simulink model "gold_mine"  (R2024b)
settings: Solver=VariableStepAuto  StartTime=0.0  StopTime=1  RelTol=1e-3
values from neighbouring files (symbols this model uses):
  Capital_expenditure = plan_4mt(:, 14)    [DCF_Model_for_Mining_Inv.m]
  discount_rate = 0.10    (= 0.1)    [DCF_Model_for_Mining_Inv.m]
  Gold_price = gold_price_matrix    [DCF_Model_for_Mining_Inv.m]
  inflation = 0.02    [DCF_Model_for_Mining_Inv.m]
  Mill1 = plan_4mt(:, 3)    [DCF_Model_for_Mining_Inv.m]
  Mill_Au_GRADE = plan_4mt(:, 4)    [DCF_Model_for_Mining_Inv.m]
  mining_cost_initial = 3.10    (= 3.1)    [DCF_Model_for_Mining_Inv.m]
  Period = plan_4mt(:, 1)    [DCF_Model_for_Mining_Inv.m]
  Recovery_rate = plan_4mt(:, 8)    [DCF_Model_for_Mining_Inv.m]
  Tax_and_royalty = plan_4mt(:, 17)    [DCF_Model_for_Mining_Inv.m]
  Tonnes = plan_4mt(:, 2)    [DCF_Model_for_Mining_Inv.m]
  Unit_processing_cost = plan_4mt(:, 10)    [DCF_Model_for_Mining_Inv.m]
undefined symbols (not defined in the file or in its folder): Stockpile_in, Stockpile_out, Waste
settings Model: Creator=eerolindholm  LastModifiedBy=eerolindholm

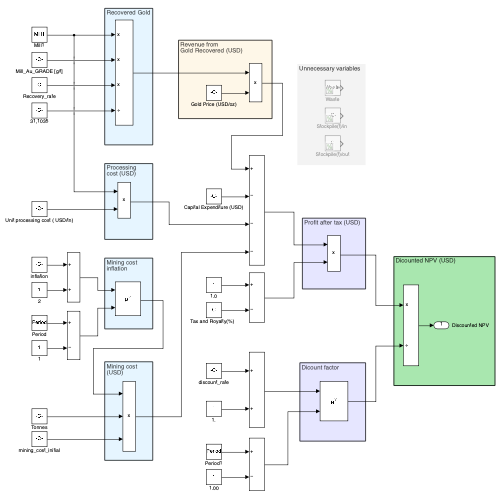
[thumbnail: Simulink's stored preview of the top-level diagram]
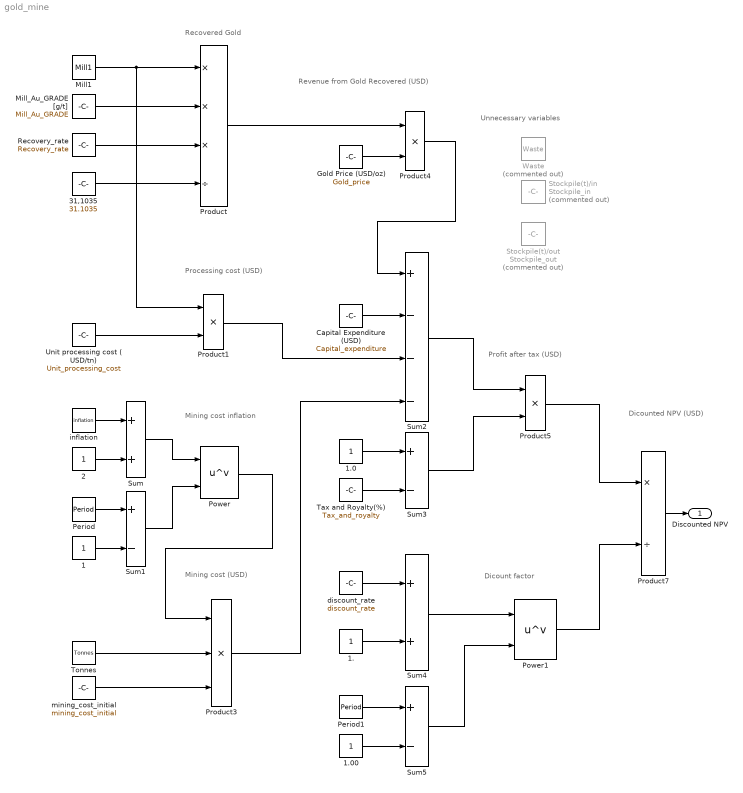
== system gold_mine ==
  note: Unnecessary variables
  note: Dicounted NPV (USD)
  note: Dicount factor
  note: Profit after tax (USD)
  note: Revenue from
      | Gold Recovered (USD)
  note: Mining cost
      | inflation
  note: Recovered Gold
  note: Processing
      | cost (USD)
  note: Mining cost
      | (USD)
  1 : Constant
  1. : Constant
  1.0 : Constant
  1.00 : Constant
  2 : Constant
  31,1035 : Constant  Value=31.1035
  Capital Expenditure (USD) : Constant  Value=Capital_expenditure
  Gold Price (USD/oz) : Constant  Value=Gold_price
  Mill1 : Constant  Value=Mill1
  Mill_Au_GRADE [g/t] : Constant  Value=Mill_Au_GRADE
  Period : Constant  Value=Period
  Period1 : Constant  Value=Period
  Power : Math  Operator=pow
  Power1 : Math  Operator=pow
  Product : Product  Inputs=***/
  Product1 : Product  Inputs=**
  Product3 : Product  Inputs=***
  Product4 : Product  Inputs=**
  Product5 : Product  Inputs=**
  Product7 : Product  Inputs=*/
  Recovery_rate : Constant  Value=Recovery_rate
  "Stockpile(t)/in " : Constant  Commented=on  Value=Stockpile_in
  Stockpile(t)/out : Constant  Commented=on  Value=Stockpile_out
  Sum : Sum
  Sum1 : Sum  Inputs=+-
  Sum2 : Sum  Inputs=+---
  Sum3 : Sum  Inputs=+-
  Sum4 : Sum
  Sum5 : Sum  Inputs=+-
  "Tax and Royalty(%)  " : Constant  Value=Tax_and_royalty
  Tonnes : Constant  Value=Tonnes
  Unit processing cost ( USD/tn) : Constant  Value=Unit_processing_cost
  Waste : Constant  Commented=on  Value=Waste
  discount_rate : Constant  Value=discount_rate
  inflation : Constant  Value=inflation
  mining_cost_initial : Constant  Value=mining_cost_initial
  Discounted NPV : Outport
  wires:
  Sum2/1 -> Product5/1
  Sum3/1 -> Product5/2
  1.0/1 -> Sum3/1
  "Tax and Royalty(%)  "/1 -> Sum3/2
  discount_rate/1 -> Sum4/1
  1./1 -> Sum4/2
  Sum5/1 -> Power1/2
  Sum4/1 -> Power1/1
  1.00/1 -> Sum5/2
  Period1/1 -> Sum5/1
  Product7/1 -> Discounted NPV/1
  Power1/1 -> Product7/2
  Product5/1 -> Product7/1
  Product3/1 -> Sum2/4
  Power/1 -> Product3/1
  Sum1/1 -> Power/2
  Period/1 -> Sum1/1
  1/1 -> Sum1/2
  2/1 -> Sum/2
  inflation/1 -> Sum/1
  Sum/1 -> Power/1
  Product1/1 -> Sum2/3
  Capital Expenditure (USD)/1 -> Sum2/2
  Product4/1 -> Sum2/1
  Gold Price (USD/oz)/1 -> Product4/2
  Product/1 -> Product4/1
  Mill_Au_GRADE [g/t]/1 -> Product/2
  Recovery_rate/1 -> Product/3
  31,1035/1 -> Product/4
  Unit processing cost ( USD/tn)/1 -> Product1/2
  mining_cost_initial/1 -> Product3/3
  Tonnes/1 -> Product3/2
  Mill1/1 -> Product/1, Product1/1
